simulink model "Speed_Controller_Test_gr3"  (Simulink 7.0)
settings: Solver=ode4  SolverMode=SingleTasking  StartTime=0.0  StopTime=252  FixedStep=0.01  RelTol=1e-3
InitFcn:
  | tempomat_para
StopFcn:
  | clear;
values from neighbouring files (symbols this model uses):
  A = 1.9    [tempomat_para.m]
  a_Fzg_max = 2    [tempomat_para.m]
  a_Fzg_min = -2    [tempomat_para.m]
  cw = 0.32    [tempomat_para.m]
  gang = [1 2 3 4]    [tempomat_para.m]
  gang_vec = [1 2 3 4]    [tempomat_para.m]
  i_anteil = 5    [tempomat_para.m]
  i_d = 3.42    [tempomat_para.m]
  i_g = [3.91 2.17 1.37 1.00]    [tempomat_para.m]
  lambda_gang = [1.3 1.25  1.17  1.05]    [tempomat_para.m]
  m_Fzg = 1400    [tempomat_para.m]
  M_mot_max = [130 149 163 170 168 166 162 158 150 139 123 80]    [tempomat_para.m]
  M_mot_min = [0 -40]    [tempomat_para.m]
  n_mot0 = 1000    [tempomat_para.m]
  n_mot_max = 1000:500:6500    [tempomat_para.m]
  n_mot_min = [1000 6500]    [tempomat_para.m]
  p_anteil = 100    [tempomat_para.m]
  r_dyn = 0.28    [tempomat_para.m]
  rho = 1.202    [tempomat_para.m]
  t_sch = 0.2    [tempomat_para.m]
  TI = [block '/TI']    [PSTI_callback.m]
  v_Fzg_ms0 = 0    [tempomat_para.m]
undefined symbols (not defined in the file or in its folder): Drossel_mat, getdatatypespecs
libraries: simulink x284, fzgbib x6
(part 15 of 19)

== system Speed_Controller_Test_gr3/Test Specification/R1 Speed Control step response/Maximum overshoot < 5 &  Steady state error < 5/Step response characteristics/Step response characteristics extraction/Extract steady state error ==
  Step response : Inport  OutDataType=sfix(16)  OutScaling=2^0
  Set point : Inport  Port=2  OutDataType=sfix(16)  OutScaling=2^0
  Subtract : Sum  Inputs=+-  OutDataType=sfix(16)  OutScaling=2^-10
  Weighted Moving Average : S-Function  FunctionName=sfix_fir  Parameters=(getdatatypespecs(OutDataType,OutScaling,DblOver,0)),[DoSatur RndMeth-1],DblOver,dolog,mgainval,(getdatatypespecs(GainDataType,GainScaling,DblOver,RadixGroup)),samptime,vinit,OutputDataTypeScalingMode,GainDataTypeScalingMode  mask(Weighted Moving Average){mgainval=0.01*ones(1,100), vinit=0.0, samptime=-1, GainDataTypeScalingMode=Inherit via internal rule, GainDataType=sfix( 16 ), MatRadixGroup=Best Precision: Matrix-wise, GainScaling=2^-10, OutputDataTypeScalingMode=Inherit via internal rule, OutDataType=sfix(16), OutScaling=2^-10, LockScale=off, RndMeth=Floor, DoSatur=off}
      mask prompts: mgainval "Weights:"; vinit "Initial condition:"; samptime "Sample time:"; GainDataTypeScalingMode "Gain data type and scaling:"; GainDataType "Parameter data type:     ex. sfix(16),  uint(8), float('single')"; MatRadixGroup "Parameter scaling mode:"; GainScaling "Parameter scaling:    Slope    ex.  2^-9"; OutputDataTypeScalingMode "Output data type and scaling:"; OutDataType "Output data type:     ex.  sfix(16),  uint(8),  float('single')"; OutScaling "Output scaling:    Slope or [Slope Bias]    ex.  2^-9"; LockScale "Lock output scaling so autoscaling tool can't change it"; RndMeth "Round toward:"; DoSatur "Saturate to max or min when overflows occur"
      mask help: Output the weighted moving average of the input.
      mask init:
      | DblOver = 0;
      | dolog = 0;
      | 
      | if MatRadixGroup == 5
      |     RadixGroup = 1; % BEST_PREC_MAT
      | elseif MatRadixGroup == 4
      |     RadixGroup = 2; % BEST_PREC_COL
      | elseif MatRadixGroup == 3
      |     RadixGroup = 3; % BEST_PREC_ROW
      | elseif MatRadixGroup == 2
      |     RadixGroup = 4; % BEST_PREC_ELE
      | else
      |     RadixGroup = 0; % BEST_PREC_OFF
      | end
      mask StyleString: edit,edit,edit,popup(Specify via dialog|Inherit via internal rule),edit,popup(Use Specified Scaling|Best Precision: Element-wise|Best Precision: Row-wise|Best Precision: Column-wise|Best Precision: Matrix-wise),edit,popup(Specify via dialog|Inherit via internal rule|Inherit via back propagation),edit,edit,checkbox,popup(Zero|Nearest|Ceiling|Floor),checkbox
      mask CallbackString: |||fixptdialog(gcbh)|fixptdialog(gcbh)|fixptdialog(gcbh)||fixptdialog(gcbh)|fixptdialog(gcbh)||||
      mask TabNameString: Main,Main,Main,Parameter data types,Parameter data types,Parameter data types,Parameter data types,Signal data types,Signal data types,Signal data types,Signal data types,Signal data types,Signal data types
      mask Display:
      | fprintf(fixpt_fir_mask_data(mgainval,'dispstr'))
      | plot(fixpt_fir_mask_data(mgainval,1),fixpt_fir_mask_data(mgainval,0))
  ss error : Outport  OutDataType=sfix(16)  OutScaling=2^0
  wires:
  Step response/1 -> Subtract/1
  Set point/1 -> Subtract/2
  Subtract/1 -> Weighted Moving Average/1
  Weighted Moving Average/1 -> ss error/1

== system Speed_Controller_Test_gr3/Test Specification/R1 Speed Control step response/Maximum overshoot < 5 &  Steady state error < 5/Step response characteristics/Step response characteristics extraction/Step time ==
  Clock : Inport  OutDataType=sfix(16)  OutScaling=2^0
  Trigger : TriggerPort
  Time : Outport  OutDataType=sfix(16)  OutScaling=2^0
  wires:
  Clock/1 -> Time/1

== system Speed_Controller_Test_gr3/Test Specification/R1 Speed Control step response/Maximum overshoot < 5 &  Steady state error < 5/Step response characteristics/Step response reset/Active if signals constant for some specified time ==
  Signal1 : Inport  OutDataType=sfix(16)  OutScaling=2^0
  Signal 2 : Inport  Port=2  OutDataType=sfix(16)  OutScaling=2^0
  Logical Operator1 : Logic  AllPortsSameDT=off  OutDataTypeMode=boolean
  Min Time : Constant  Value=10  OutDataType=sfix(16)  OutScaling=2^0
  MinMax : MinMax  Inputs=2  OutDataType=sfix(16)  OutScaling=2^0
  Relational Operator2 : RelationalOperator  Operator=<=  LogicOutDataTypeMode=boolean
  Switch : Switch  Criteria=u2 ~= 0
  Time since signal constant : Subsystem  TreatAsAtomicUnit=on  mask(Feature extraction block){RT=0.0001}
      mask prompts: RT "Relative tolerance in %"
      mask help: Detect if the signal value is constant (using the last two signal values) allowing for a user-defined relative deviation
      mask CallbackString:
      | if or( (str2double(get_param(gcb,'RT')) < 0), (str2double(get_param(gcb,'RT')) > 100))
      |     error(['Relative tolerance value (' get_param(gcb,'RT') ') out of range. Please give a value between 0 and 100.']);
      | else
      |     set_param([gcb '/Detect constant/Relative tolerance/Relative Tolerance'],'Value',get_param(gcb,'RT'));
      |     set_param([gcb '/Detect constant'],'RT',get_param(gcb,'RT'));
      | end
  Time since signal constant1 : Subsystem  TreatAsAtomicUnit=on  mask(Feature extraction block){RT=0.0001}
      mask prompts: RT "Relative tolerance in %"
      mask help: Detect if the signal value is constant (using the last two signal values) allowing for a user-defined relative deviation
      mask CallbackString:
      | if or( (str2double(get_param(gcb,'RT')) < 0), (str2double(get_param(gcb,'RT')) > 100))
      |     error(['Relative tolerance value (' get_param(gcb,'RT') ') out of range. Please give a value between 0 and 100.']);
      | else
      |     set_param([gcb '/Detect constant/Relative tolerance/Relative Tolerance'],'Value',get_param(gcb,'RT'));
      |     set_param([gcb '/Detect constant'],'RT',get_param(gcb,'RT'));
      | end
  Zero : Constant  Value=0  OutDataType=sfix(16)  OutScaling=2^0
  Constant signals : Outport  OutDataType=sfix(16)  OutScaling=2^0
  wires:
  Signal1/1 -> Time since signal constant/1(Signal)
  Signal 2/1 -> Time since signal constant1/1(Signal)
  Relational Operator2/1 -> Constant signals/1
  Min Time/1 -> Relational Operator2/1
  Switch/1 -> Relational Operator2/2
  Time since signal constant1/2(Feature) -> MinMax/2
  Time since signal constant/2(Feature) -> MinMax/1
  Time since signal constant/1(Trigger) -> Logical Operator1/1
  Time since signal constant1/1(Trigger) -> Logical Operator1/2
  MinMax/1 -> Switch/1
  Logical Operator1/1 -> Switch/2
  Zero/1 -> Switch/3

== system Speed_Controller_Test_gr3/Test Specification/R1 Speed Control step response/Maximum overshoot < 5 &  Steady state error < 5/Step response characteristics/Step response reset/Step detection ==
  Signal : Inport  OutDataType=sfix(16)  OutScaling=2^0
  Abs : Abs
  Add : Sum  Inputs=+-  OutDataType=sfix(16)  OutScaling=2^-10
  Clock : Clock
      settings: Decimation=10
  Memory : Memory
  Min step size : Constant  Value=10  OutDataType=sfix(16)  OutScaling=2^0
  Relational Operator : RelationalOperator  LogicOutDataTypeMode=boolean
  Switch : Switch  Criteria=u2 > Threshold
  Step : Outport  OutDataType=sfix(16)  OutScaling=2^0
  wires:
  Add/1 -> Abs/1
  Relational Operator/1 -> Step/1
  Min step size/1 -> Relational Operator/2
  Abs/1 -> Relational Operator/1
  Signal/1 -> Memory/1, Switch/3, Add/1
  Clock/1 -> Switch/2
  Memory/1 -> Switch/1
  Switch/1 -> Add/2

== system Speed_Controller_Test_gr3/Test Specification/R1 Speed Control step response/Maximum overshoot < 5 &  Steady state error < 5/Step response characteristics/Step response trigger/Active if signals constant for some specified time ==
  Signal1 : Inport  OutDataType=sfix(16)  OutScaling=2^0
  Signal 2 : Inport  Port=2  OutDataType=sfix(16)  OutScaling=2^0
  Logical Operator1 : Logic  AllPortsSameDT=off  OutDataTypeMode=boolean
  Min Time : Constant  Value=10  OutDataType=sfix(16)  OutScaling=2^0
  MinMax : MinMax  Inputs=2  OutDataType=sfix(16)  OutScaling=2^0
  Relational Operator2 : RelationalOperator  Operator=<=  LogicOutDataTypeMode=boolean
  Switch : Switch  Criteria=u2 ~= 0
  Time since signal constant : Subsystem  TreatAsAtomicUnit=on  mask(Feature extraction block){RT=0.001}
      mask prompts: RT "Relative tolerance in %"
      mask help: Detect if the signal value is constant (using the last two signal values) allowing for a user-defined relative deviation
      mask CallbackString:
      | if or( (str2double(get_param(gcb,'RT')) < 0), (str2double(get_param(gcb,'RT')) > 100))
      |     error(['Relative tolerance value (' get_param(gcb,'RT') ') out of range. Please give a value between 0 and 100.']);
      | else
      |     set_param([gcb '/Detect constant/Relative tolerance/Relative Tolerance'],'Value',get_param(gcb,'RT'));
      |     set_param([gcb '/Detect constant'],'RT',get_param(gcb,'RT'));
      | end
  Time since signal constant1 : Subsystem  TreatAsAtomicUnit=on  mask(Feature extraction block){RT=0.001}
      mask prompts: RT "Relative tolerance in %"
      mask help: Detect if the signal value is constant (using the last two signal values) allowing for a user-defined relative deviation
      mask CallbackString:
      | if or( (str2double(get_param(gcb,'RT')) < 0), (str2double(get_param(gcb,'RT')) > 100))
      |     error(['Relative tolerance value (' get_param(gcb,'RT') ') out of range. Please give a value between 0 and 100.']);
      | else
      |     set_param([gcb '/Detect constant/Relative tolerance/Relative Tolerance'],'Value',get_param(gcb,'RT'));
      |     set_param([gcb '/Detect constant'],'RT',get_param(gcb,'RT'));
      | end
  Zero : Constant  Value=0  OutDataType=sfix(16)  OutScaling=2^0
  Constant signals : Outport  OutDataType=sfix(16)  OutScaling=2^0
  wires:
  Signal1/1 -> Time since signal constant/1(Signal)
  Signal 2/1 -> Time since signal constant1/1(Signal)
  Relational Operator2/1 -> Constant signals/1
  Min Time/1 -> Relational Operator2/1
  Switch/1 -> Relational Operator2/2
  Time since signal constant1/2(Feature) -> MinMax/2
  Time since signal constant/2(Feature) -> MinMax/1
  Time since signal constant/1(Trigger) -> Logical Operator1/1
  Time since signal constant1/1(Trigger) -> Logical Operator1/2
  MinMax/1 -> Switch/1
  Logical Operator1/1 -> Switch/2
  Zero/1 -> Switch/3

== system Speed_Controller_Test_gr3/Test Specification/R1 Speed Control step response/Maximum overshoot < 5 &  Steady state error < 5/Step response characteristics/Step response trigger/Compare To Constant ==
  u : Inport  OutDataType=sfix(16)  OutScaling=2^0
  Compare : RelationalOperator  Operator=<=  LogicOutDataTypeMode=Specify via dialog  ZeroCross=off  InputSameDT=on
  Constant : Constant  Value=const  OutDataType=sfix(16)  OutScaling=1
  y : Outport  OutDataType=sfix(16)  OutScaling=2^0
  wires:
  Compare/1 -> y/1
  Constant/1 -> Compare/2
  u/1 -> Compare/1

== system Speed_Controller_Test_gr3/Test Specification/R1 Speed Control step response/Maximum overshoot < 5 &  Steady state error < 5/Step response characteristics/Step response trigger/Detect increase ==
  Signal : Inport  OutDataType=sfix(16)  OutScaling=2^0
  Clock : Clock
      settings: Decimation=10
  Memory : Memory
  Relational Operator : RelationalOperator  Operator=>  LogicOutDataTypeMode=Specify via dialog
  Switch : Switch  Criteria=u2 > Threshold
  Increase : Outport  OutDataType=sfix(16)  OutScaling=2^0
  wires:
  Switch/1 -> Relational Operator/2
  Memory/1 -> Switch/1
  Clock/1 -> Switch/2
  Relational Operator/1 -> Increase/1
  Signal/1 -> Switch/3, Memory/1, Relational Operator/1

== system Speed_Controller_Test_gr3/Test Specification/R2 Speed Control velocity restoration time after simple  acceleration/deceleration/CC active + no target & Speed Control active & step of V_Des = |1|  with time periods >= 7s/PS/TI/Delays1 ==
  In1 : Inport  OutDataType=sfix(16)  OutScaling=2^0
  Delay : Constant  Value=0  OutDataType=sfix(16)  OutScaling=2^0
  Integer Delay : S-Function  FunctionName=sfix_udelay  Parameters=samptime,vinit,NumDelays,1,1,0  mask(Integer Delay){vinit=0.0, samptime=-1, NumDelays=15}
      mask prompts: vinit "Initial condition:"; samptime "Sample time:"; NumDelays "Number of delays:"
      mask help: Delay a signal N sample periods.
      mask init:
      | if isempty(NumDelays)
      |    NumDelays = 1;
      | end
      mask Display: fprintf(' %d\nZ   ',-1*(NumDelays))
  Switch : Switch  Criteria=u2 ~= 0
  Out1 : Outport  OutDataType=sfix(16)  OutScaling=2^0
  wires:
  Switch/1 -> Out1/1
  In1/1 -> Switch/3, Integer Delay/1
  Delay/1 -> Switch/2
  Integer Delay/1 -> Switch/1

== system Speed_Controller_Test_gr3/Test Specification/R2 Speed Control velocity restoration time after simple  acceleration/deceleration/CC active + no target & Speed Control active & step of V_Des = |1|  with time periods >= 7s/PS/TI/Delays2 ==
  In1 : Inport  OutDataType=sfix(16)  OutScaling=2^0
  Delay : Constant  Value=0  OutDataType=sfix(16)  OutScaling=2^0
  Integer Delay : S-Function  FunctionName=sfix_udelay  Parameters=samptime,vinit,NumDelays,1,1,0  mask(Integer Delay){vinit=0.0, samptime=-1, NumDelays=15}
      mask prompts: vinit "Initial condition:"; samptime "Sample time:"; NumDelays "Number of delays:"
      mask help: Delay a signal N sample periods.
      mask init:
      | if isempty(NumDelays)
      |    NumDelays = 1;
      | end
      mask Display: fprintf(' %d\nZ   ',-1*(NumDelays))
  Switch : Switch  Criteria=u2 ~= 0
  Out1 : Outport  OutDataType=sfix(16)  OutScaling=2^0
  wires:
  Switch/1 -> Out1/1
  In1/1 -> Switch/3, Integer Delay/1
  Delay/1 -> Switch/2
  Integer Delay/1 -> Switch/1

== system Speed_Controller_Test_gr3/Test Specification/R2 Speed Control velocity restoration time after simple  acceleration/deceleration/CC active + no target & Speed Control active & step of V_Des = |1|  with time periods >= 7s/PS/TI/Delays3 ==
  In1 : Inport  OutDataType=sfix(16)  OutScaling=2^0
  Delay : Constant  Value=0  OutDataType=sfix(16)  OutScaling=2^0
  Integer Delay : S-Function  FunctionName=sfix_udelay  Parameters=samptime,vinit,NumDelays,1,1,0  mask(Integer Delay){vinit=0.0, samptime=-1, NumDelays=15}
      mask prompts: vinit "Initial condition:"; samptime "Sample time:"; NumDelays "Number of delays:"
      mask help: Delay a signal N sample periods.
      mask init:
      | if isempty(NumDelays)
      |    NumDelays = 1;
      | end
      mask Display: fprintf(' %d\nZ   ',-1*(NumDelays))
  Switch : Switch  Criteria=u2 ~= 0
  Out1 : Outport  OutDataType=sfix(16)  OutScaling=2^0
  wires:
  Switch/1 -> Out1/1
  In1/1 -> Switch/3, Integer Delay/1
  Delay/1 -> Switch/2
  Integer Delay/1 -> Switch/1

== system Speed_Controller_Test_gr3/Test Specification/R2 Speed Control velocity restoration time after simple  acceleration/deceleration/CC active + no target & Speed Control active & step of V_Des = |1|  with time periods >= 7s/PS/TID/Hold ==
  " " : Inport  OutDataType=sfix(16)  OutScaling=2^0
  "    " : Inport  Port=2  OutDataType=sfix(16)  OutScaling=2^0
  Memory : Memory  Orientation=left
  Switch : Switch  Criteria=u2 ~= 0
  "  " : Outport  OutDataType=sfix(16)  OutScaling=2^0
  wires:
  Memory/1 -> Switch/3
  Switch/1 -> Memory/1, "  "/1
  "    "/1 -> Switch/1
  " "/1 -> Switch/2

== system Speed_Controller_Test_gr3/Test Specification/R2 Speed Control velocity restoration time after simple  acceleration/deceleration/CC active + no target & Speed Control active & step of V_Des = |1|  with time periods >= 7s/Step with step size=|1|  and time periods >= 6s detection/Step detection/Active if signals constant for some specified time ==
  Signal 2 : Inport  OutDataType=sfix(16)  OutScaling=2^0
  Min Time : Constant  Value=6  OutDataType=sfix(16)  OutScaling=2^0
  Relational Operator2 : RelationalOperator  Operator=<=  LogicOutDataTypeMode=boolean
  Switch : Switch  Criteria=u2 ~= 0
  Time since signal constant1 : Subsystem  TreatAsAtomicUnit=on  mask(Feature extraction block){RT=0.0001}
      mask prompts: RT "Relative tolerance in %"
      mask help: Detect if the signal value is constant (using the last two signal values) allowing for a user-defined relative deviation
      mask CallbackString:
      | if or( (str2double(get_param(gcb,'RT')) < 0), (str2double(get_param(gcb,'RT')) > 100))
      |     error(['Relative tolerance value (' get_param(gcb,'RT') ') out of range. Please give a value between 0 and 100.']);
      | else
      |     set_param([gcb '/Detect constant/Relative tolerance/Relative Tolerance'],'Value',get_param(gcb,'RT'));
      |     set_param([gcb '/Detect constant'],'RT',get_param(gcb,'RT'));
      | end
  Zero : Constant  Value=0  OutDataType=sfix(16)  OutScaling=2^0
  Constant signals : Outport  OutDataType=sfix(16)  OutScaling=2^0
  wires:
  Signal 2/1 -> Time since signal constant1/1(Signal)
  Relational Operator2/1 -> Constant signals/1
  Min Time/1 -> Relational Operator2/1
  Switch/1 -> Relational Operator2/2
  Time since signal constant1/2(Feature) -> Switch/1
  Time since signal constant1/1(Trigger) -> Switch/2
  Zero/1 -> Switch/3

== system Speed_Controller_Test_gr3/Test Specification/R2 Speed Control velocity restoration time after simple  acceleration/deceleration/CC active + no target & Speed Control active & step of V_Des = |1|  with time periods >= 7s/Step with step size=|1|  and time periods >= 6s detection/Step detection/Step detection ==
  Signal : Inport  OutDataType=sfix(16)  OutScaling=2^0
  Abs : Abs
  Add : Sum  Inputs=+-  OutDataType=sfix(16)  OutScaling=2^-10
  Clock : Clock
      settings: Decimation=10
  Memory : Memory
  Relational Operator : RelationalOperator  Operator===  LogicOutDataTypeMode=boolean
  Step size : Constant  OutDataType=sfix(16)  OutScaling=2^0
  Switch : Switch  Criteria=u2 > Threshold
  Step : Outport  OutDataType=sfix(16)  OutScaling=2^0
  wires:
  Add/1 -> Abs/1
  Step size/1 -> Relational Operator/2
  Abs/1 -> Relational Operator/1
  Signal/1 -> Memory/1, Switch/3, Add/1
  Clock/1 -> Switch/2
  Memory/1 -> Switch/1
  Switch/1 -> Add/2
  Relational Operator/1 -> Step/1

== system Speed_Controller_Test_gr3/Test Specification/R2 Speed Control velocity restoration time after simple  acceleration/deceleration/after (6 seconds)  |V_Des-V_Vhcl <= 1.4|/PAS1/Delay bus signals/AD delay ==
  In1 : Inport  OutDataType=sfix(16)  OutScaling=2^0
  Delay : Constant  Value=0  OutDataType=sfix(16)  OutScaling=2^0
  Integer Delay : S-Function  FunctionName=sfix_udelay  Parameters=samptime,vinit,NumDelays,1,1,0  mask(Integer Delay){vinit=0.0, samptime=-1, NumDelays=15}
      mask prompts: vinit "Initial condition:"; samptime "Sample time:"; NumDelays "Number of delays:"
      mask help: Delay a signal N sample periods.
      mask init:
      | if isempty(NumDelays)
      |    NumDelays = 1;
      | end
      mask Display: fprintf(' %d\nZ   ',-1*(NumDelays))
  Switch : Switch  Criteria=u2 ~= 0
  Out1 : Outport  OutDataType=sfix(16)  OutScaling=2^0
  wires:
  Switch/1 -> Out1/1
  In1/1 -> Switch/3, Integer Delay/1
  Delay/1 -> Switch/2
  Integer Delay/1 -> Switch/1

== system Speed_Controller_Test_gr3/Test Specification/R2 Speed Control velocity restoration time after simple  acceleration/deceleration/after (6 seconds)  |V_Des-V_Vhcl <= 1.4|/PAS1/Delay bus signals/ELL delay ==
  In1 : Inport  OutDataType=sfix(16)  OutScaling=2^0
  Delay : Constant  Value=0  OutDataType=sfix(16)  OutScaling=2^0
  Integer Delay : S-Function  FunctionName=sfix_udelay  Parameters=samptime,vinit,NumDelays,1,1,0  mask(Integer Delay){vinit=0.0, samptime=-1, NumDelays=15}
      mask prompts: vinit "Initial condition:"; samptime "Sample time:"; NumDelays "Number of delays:"
      mask help: Delay a signal N sample periods.
      mask init:
      | if isempty(NumDelays)
      |    NumDelays = 1;
      | end
      mask Display: fprintf(' %d\nZ   ',-1*(NumDelays))
  Switch : Switch  Criteria=u2 ~= 0
  Out1 : Outport  OutDataType=sfix(16)  OutScaling=2^0
  wires:
  Switch/1 -> Out1/1
  In1/1 -> Switch/3, Integer Delay/1
  Delay/1 -> Switch/2
  Integer Delay/1 -> Switch/1

== system Speed_Controller_Test_gr3/Test Specification/R2 Speed Control velocity restoration time after simple  acceleration/deceleration/after (6 seconds)  |V_Des-V_Vhcl <= 1.4|/PAS1/Delay bus signals/EUL delay ==
  In1 : Inport  OutDataType=sfix(16)  OutScaling=2^0
  Delay : Constant  Value=0  OutDataType=sfix(16)  OutScaling=2^0
  Integer Delay : S-Function  FunctionName=sfix_udelay  Parameters=samptime,vinit,NumDelays,1,1,0  mask(Integer Delay){vinit=0.0, samptime=-1, NumDelays=15}
      mask prompts: vinit "Initial condition:"; samptime "Sample time:"; NumDelays "Number of delays:"
      mask help: Delay a signal N sample periods.
      mask init:
      | if isempty(NumDelays)
      |    NumDelays = 1;
      | end
      mask Display: fprintf(' %d\nZ   ',-1*(NumDelays))
  Switch : Switch  Criteria=u2 ~= 0
  Out1 : Outport  OutDataType=sfix(16)  OutScaling=2^0
  wires:
  Integer Delay/1 -> Switch/1
  Delay/1 -> Switch/2
  In1/1 -> Integer Delay/1, Switch/3
  Switch/1 -> Out1/1

== system Speed_Controller_Test_gr3/Test Specification/R2 Speed Control velocity restoration time after simple  acceleration/deceleration/after (6 seconds)  |V_Des-V_Vhcl <= 1.4|/PAS1/none - pass - fail/Arbitration ==
  Pass : Inport  OutDataType=sfix(16)  OutScaling=2^0
  Fail1 : Inport  Port=2  OutDataType=sfix(16)  OutScaling=2^0
  Fail2 : Inport  Port=3  OutDataType=sfix(16)  OutScaling=2^0
  Fail3 : Inport  Port=4  OutDataType=sfix(16)  OutScaling=2^0
  Fail4 : Inport  Port=5  OutDataType=sfix(16)  OutScaling=2^0
  Delay P F1 F3 : Inport  Port=6  OutDataType=sfix(16)  OutScaling=2^0
  Delay F2 : Inport  Port=7  OutDataType=sfix(16)  OutScaling=2^0
  Delay F4 : Inport  Port=8  OutDataType=sfix(16)  OutScaling=2^0
  Max delay : Inport  Port=9  OutDataType=sfix(16)  OutScaling=2^0
  Verdict identification : Subsystem
  Verdict selection : Subsystem
  Verdict : Outport  OutDataType=sfix(16)  OutScaling=2^0
  Delay : Outport  Port=2  OutDataType=sfix(16)  OutScaling=2^0
  wires:
  Verdict selection/2(Delay) -> Delay/1
  Verdict selection/1(Verdict) -> Verdict/1
  Max delay/1 -> Verdict selection/6(Max delay)
  Verdict identification/2(V2) -> Verdict selection/2(V2)
  Verdict identification/1(V1) -> Verdict selection/1(V1)
  Delay F4/1 -> Verdict selection/5(Delay F4)
  Delay F2/1 -> Verdict selection/4(Delay F2)
  Delay P F1 F3/1 -> Verdict selection/3(Delay P F1 F3)
  Fail4/1 -> Verdict identification/5(Fail4)
  Fail3/1 -> Verdict identification/4(Fail3)
  Fail2/1 -> Verdict identification/3(Fail2)
  Fail1/1 -> Verdict identification/2(Fail1)
  Pass/1 -> Verdict identification/1(Pass)

== system Speed_Controller_Test_gr3/Test Specification/R2 Speed Control velocity restoration time after simple  acceleration/deceleration/after (6 seconds)  |V_Des-V_Vhcl <= 1.4|/PAS1/none - pass - fail/Compute delay ==
  Max Delay : Inport  OutDataType=sfix(16)  OutScaling=2^0
  R AND : Inport  Port=2  OutDataType=sfix(16)  OutScaling=2^0
  Clock : Clock
      settings: Decimation=10
  Clock1 : Clock
      settings: Decimation=10
  Divide : Product  Inputs=/*  OutDataType=sfix(16)  OutScaling=2^-10
  Hold1 : Subsystem  TreatAsAtomicUnit=on
      mask Display: patch(-0.31+[0.4 0.46 0.46 0.54 0.54 0.6 0.6 0.55 0.55 0.45 0.45 0.4],-0.19+[0.85 0.85 0.95 0.95 0.85 0.85 0.87 0.87 0.96 0.96 0.87 0.87],[0 0 0]);
  SimStepSize : Constant  Value=0.01  OutDataType=sfix(16)  OutScaling=2^0
  Subtract : Sum  Inputs=-+  OutDataType=sfix(16)  OutScaling=2^-10
  Subtract1 : Sum  Inputs=+-  OutDataType=sfix(16)  OutScaling=2^-10
  Delay : Outport  OutDataType=sfix(16)  OutScaling=2^0
  wires:
  Divide/1 -> Delay/1
  Max Delay/1 -> Subtract/1
  SimStepSize/1 -> Divide/1
  Clock/1 -> Hold1/2("    ")
  Subtract/1 -> Subtract1/2
  Subtract1/1 -> Divide/2
  Clock1/1 -> Subtract1/1
  Hold1/1("  ") -> Subtract/2
  R AND/1 -> Hold1/1(" ")

== system Speed_Controller_Test_gr3/Test Specification/R2 Speed Control velocity restoration time after simple  acceleration/deceleration/after (6 seconds)  |V_Des-V_Vhcl <= 1.4|/PAS1/none - pass - fail/Compute delay1 ==
  Max Delay : Inport  OutDataType=sfix(16)  OutScaling=2^0
  R AND/z : Inport  Port=2  OutDataType=sfix(16)  OutScaling=2^0
  Add : Sum  OutDataType=sfix(16)  OutScaling=2^-10
  Clock : Clock
      settings: Decimation=10
  Clock1 : Clock
      settings: Decimation=10
  Divide : Product  Inputs=/*  OutDataType=sfix(16)  OutScaling=2^-10
  Hold1 : Subsystem  TreatAsAtomicUnit=on
      mask Display: patch(-0.31+[0.4 0.46 0.46 0.54 0.54 0.6 0.6 0.55 0.55 0.45 0.45 0.4],-0.19+[0.85 0.85 0.95 0.95 0.85 0.85 0.87 0.87 0.96 0.96 0.87 0.87],[0 0 0]);
  SimStepSize : Constant  Value=0.01  OutDataType=sfix(16)  OutScaling=2^0
  Subtract : Sum  Inputs=-+  OutDataType=sfix(16)  OutScaling=2^-10
  Subtract1 : Sum  Inputs=+-  OutDataType=sfix(16)  OutScaling=2^-10
  Unit : Constant  OutDataType=sfix(16)  OutScaling=2^0
  Delay : Outport  OutDataType=sfix(16)  OutScaling=2^0
  wires:
  Divide/1 -> Add/2
  Unit/1 -> Add/1
  Max Delay/1 -> Subtract/1
  SimStepSize/1 -> Divide/1
  Clock/1 -> Hold1/2("    ")
  Subtract/1 -> Subtract1/2
  Subtract1/1 -> Divide/2
  Clock1/1 -> Subtract1/1
  Hold1/1("  ") -> Subtract/2
  R AND/z/1 -> Hold1/1(" ")
  Add/1 -> Delay/1

== system Speed_Controller_Test_gr3/Test Specification/R2 Speed Control velocity restoration time after simple  acceleration/deceleration/after (6 seconds)  |V_Des-V_Vhcl <= 1.4|/PAS1/none - pass - fail/Compute delay2 ==
  Max Delay : Inport  OutDataType=sfix(16)  OutScaling=2^0
  Rp & NOT(Ra) : Inport  Port=2  OutDataType=sfix(16)  OutScaling=2^0
  Clock : Clock
      settings: Decimation=10
  Clock1 : Clock
      settings: Decimation=10
  Divide : Product  Inputs=/*  OutDataType=sfix(16)  OutScaling=2^-10
  Hold1 : Subsystem  TreatAsAtomicUnit=on
      mask Display: patch(-0.31+[0.4 0.46 0.46 0.54 0.54 0.6 0.6 0.55 0.55 0.45 0.45 0.4],-0.19+[0.85 0.85 0.95 0.95 0.85 0.85 0.87 0.87 0.96 0.96 0.87 0.87],[0 0 0]);
  SimStepSize : Constant  Value=0.01  OutDataType=sfix(16)  OutScaling=2^0
  Subtract : Sum  Inputs=-+  OutDataType=sfix(16)  OutScaling=2^-10
  Subtract1 : Sum  Inputs=+-  OutDataType=sfix(16)  OutScaling=2^-10
  Delay : Outport  OutDataType=sfix(16)  OutScaling=2^0
  wires:
  Divide/1 -> Delay/1
  Rp & NOT(Ra)/1 -> Hold1/1(" ")
  Hold1/1("  ") -> Subtract/2
  Clock1/1 -> Subtract1/1
  Subtract1/1 -> Divide/2
  Subtract/1 -> Subtract1/2
  Clock/1 -> Hold1/2("    ")
  SimStepSize/1 -> Divide/1
  Max Delay/1 -> Subtract/1

== system Speed_Controller_Test_gr3/Test Specification/R2 Speed Control velocity restoration time after simple  acceleration/deceleration/after (6 seconds)  |V_Des-V_Vhcl <= 1.4|/PAS1/none - pass - fail/Hold R AND1 ==
  " " : Inport  OutDataType=sfix(16)  OutScaling=2^0
  "    " : Inport  Port=2  OutDataType=sfix(16)  OutScaling=2^0
  Memory : Memory  Orientation=left
  Switch : Switch  Criteria=u2 ~= 0
  "  " : Outport  OutDataType=sfix(16)  OutScaling=2^0
  wires:
  Memory/1 -> Switch/3
  Switch/1 -> Memory/1, "  "/1
  "    "/1 -> Switch/1
  " "/1 -> Switch/2

== system Speed_Controller_Test_gr3/Test Specification/R2 Speed Control velocity restoration time after simple  acceleration/deceleration/after (6 seconds)  |V_Des-V_Vhcl <= 1.4|/PAS1/none - pass - fail/Hold R AND2 ==
  " " : Inport  OutDataType=sfix(16)  OutScaling=2^0
  "    " : Inport  Port=2  OutDataType=sfix(16)  OutScaling=2^0
  Memory : Memory  Orientation=left
  Switch : Switch  Criteria=u2 ~= 0
  "  " : Outport  OutDataType=sfix(16)  OutScaling=2^0
  wires:
  Memory/1 -> Switch/3
  Switch/1 -> Memory/1, "  "/1
  "    "/1 -> Switch/1
  " "/1 -> Switch/2

== system Speed_Controller_Test_gr3/Test Specification/R2 Speed Control velocity restoration time after simple  acceleration/deceleration/after (6 seconds)  |V_Des-V_Vhcl <= 1.4|/PAS1/none - pass - fail/Hold R AND3 ==
  " " : Inport  OutDataType=sfix(16)  OutScaling=2^0
  "    " : Inport  Port=2  OutDataType=sfix(16)  OutScaling=2^0
  Memory : Memory  Orientation=left
  Switch : Switch  Criteria=u2 ~= 0
  "  " : Outport  OutDataType=sfix(16)  OutScaling=2^0
  wires:
  " "/1 -> Switch/2
  "    "/1 -> Switch/1
  Switch/1 -> "  "/1, Memory/1
  Memory/1 -> Switch/3

== system Speed_Controller_Test_gr3/Test Specification/R2 Speed Control velocity restoration time after simple  acceleration/deceleration/after (6 seconds)  |V_Des-V_Vhcl <= 1.4|/PAS1/none - pass - fail/Hold1 ==
  " " : Inport  OutDataType=sfix(16)  OutScaling=2^0
  "    " : Inport  Port=2  OutDataType=sfix(16)  OutScaling=2^0
  Memory : Memory  Orientation=left
  Switch : Switch  Criteria=u2 ~= 0
  "  " : Outport  OutDataType=sfix(16)  OutScaling=2^0
  wires:
  Memory/1 -> Switch/3
  Switch/1 -> Memory/1, "  "/1
  "    "/1 -> Switch/1
  " "/1 -> Switch/2

== system Speed_Controller_Test_gr3/Test Specification/R2 Speed Control velocity restoration time after simple  acceleration/deceleration/after (6 seconds)  |V_Des-V_Vhcl <= 1.4|/PAS1/none - pass - fail/Hold2 ==
  " " : Inport  OutDataType=sfix(16)  OutScaling=2^0
  "    " : Inport  Port=2  OutDataType=sfix(16)  OutScaling=2^0
  Memory : Memory  Orientation=left
  Switch : Switch  Criteria=u2 ~= 0
  "  " : Outport  OutDataType=sfix(16)  OutScaling=2^0
  wires:
  Memory/1 -> Switch/3
  Switch/1 -> Memory/1, "  "/1
  "    "/1 -> Switch/1
  " "/1 -> Switch/2

== system Speed_Controller_Test_gr3/Test Specification/R2 Speed Control velocity restoration time after simple  acceleration/deceleration/after (6 seconds)  |V_Des-V_Vhcl <= 1.4|/PAS1/none - pass - fail/Hold3 ==
  " " : Inport  OutDataType=sfix(16)  OutScaling=2^0
  "    " : Inport  Port=2  OutDataType=sfix(16)  OutScaling=2^0
  Memory : Memory  Orientation=left
  Switch : Switch  Criteria=u2 ~= 0
  "  " : Outport  OutDataType=sfix(16)  OutScaling=2^0
  wires:
  " "/1 -> Switch/2
  "    "/1 -> Switch/1
  Switch/1 -> "  "/1, Memory/1
  Memory/1 -> Switch/3

== system Speed_Controller_Test_gr3/Test Specification/R2 Speed Control velocity restoration time after simple  acceleration/deceleration/after (6 seconds)  |V_Des-V_Vhcl <= 1.4|/PAS1/none - pass - fail/Hold4 ==
  " " : Inport  OutDataType=sfix(16)  OutScaling=2^0
  "    " : Inport  Port=2  OutDataType=sfix(16)  OutScaling=2^0
  Memory : Memory  Orientation=left
  Switch : Switch  Criteria=u2 ~= 0
  "  " : Outport  OutDataType=sfix(16)  OutScaling=2^0
  wires:
  Memory/1 -> Switch/3
  Switch/1 -> Memory/1, "  "/1
  "    "/1 -> Switch/1
  " "/1 -> Switch/2

== system Speed_Controller_Test_gr3/Test Specification/R2 Speed Control velocity restoration time after simple  acceleration/deceleration/after (6 seconds)  |V_Des-V_Vhcl <= 1.4|/PAS1/none - pass - fail/Hold5 ==
  " " : Inport  OutDataType=sfix(16)  OutScaling=2^0
  "    " : Inport  Port=2  OutDataType=sfix(16)  OutScaling=2^0
  Memory : Memory  Orientation=left
  Switch : Switch  Criteria=u2 ~= 0
  "  " : Outport  OutDataType=sfix(16)  OutScaling=2^0
  wires:
  " "/1 -> Switch/2
  "    "/1 -> Switch/1
  Switch/1 -> "  "/1, Memory/1
  Memory/1 -> Switch/3

== system Speed_Controller_Test_gr3/Test Specification/R2 Speed Control velocity restoration time after simple  acceleration/deceleration/after (6 seconds)  |V_Des-V_Vhcl <= 1.4|/PAS2/Delay bus signals/AD delay ==
  In1 : Inport  OutDataType=sfix(16)  OutScaling=2^0
  Delay : Constant  Value=0  OutDataType=sfix(16)  OutScaling=2^0
  Integer Delay : S-Function  FunctionName=sfix_udelay  Parameters=samptime,vinit,NumDelays,1,1,0  mask(Integer Delay){vinit=0.0, samptime=-1, NumDelays=15}
      mask prompts: vinit "Initial condition:"; samptime "Sample time:"; NumDelays "Number of delays:"
      mask help: Delay a signal N sample periods.
      mask init:
      | if isempty(NumDelays)
      |    NumDelays = 1;
      | end
      mask Display: fprintf(' %d\nZ   ',-1*(NumDelays))
  Switch : Switch  Criteria=u2 ~= 0
  Out1 : Outport  OutDataType=sfix(16)  OutScaling=2^0
  wires:
  Switch/1 -> Out1/1
  In1/1 -> Switch/3, Integer Delay/1
  Delay/1 -> Switch/2
  Integer Delay/1 -> Switch/1

== system Speed_Controller_Test_gr3/Test Specification/R2 Speed Control velocity restoration time after simple  acceleration/deceleration/after (6 seconds)  |V_Des-V_Vhcl <= 1.4|/PAS2/Delay bus signals/ELL delay ==
  In1 : Inport  OutDataType=sfix(16)  OutScaling=2^0
  Delay : Constant  Value=0  OutDataType=sfix(16)  OutScaling=2^0
  Integer Delay : S-Function  FunctionName=sfix_udelay  Parameters=samptime,vinit,NumDelays,1,1,0  mask(Integer Delay){vinit=0.0, samptime=-1, NumDelays=15}
      mask prompts: vinit "Initial condition:"; samptime "Sample time:"; NumDelays "Number of delays:"
      mask help: Delay a signal N sample periods.
      mask init:
      | if isempty(NumDelays)
      |    NumDelays = 1;
      | end
      mask Display: fprintf(' %d\nZ   ',-1*(NumDelays))
  Switch : Switch  Criteria=u2 ~= 0
  Out1 : Outport  OutDataType=sfix(16)  OutScaling=2^0
  wires:
  Switch/1 -> Out1/1
  In1/1 -> Switch/3, Integer Delay/1
  Delay/1 -> Switch/2
  Integer Delay/1 -> Switch/1

== system Speed_Controller_Test_gr3/Test Specification/R2 Speed Control velocity restoration time after simple  acceleration/deceleration/after (6 seconds)  |V_Des-V_Vhcl <= 1.4|/PAS2/Delay bus signals/EUL delay ==
  In1 : Inport  OutDataType=sfix(16)  OutScaling=2^0
  Delay : Constant  Value=0  OutDataType=sfix(16)  OutScaling=2^0
  Integer Delay : S-Function  FunctionName=sfix_udelay  Parameters=samptime,vinit,NumDelays,1,1,0  mask(Integer Delay){vinit=0.0, samptime=-1, NumDelays=15}
      mask prompts: vinit "Initial condition:"; samptime "Sample time:"; NumDelays "Number of delays:"
      mask help: Delay a signal N sample periods.
      mask init:
      | if isempty(NumDelays)
      |    NumDelays = 1;
      | end
      mask Display: fprintf(' %d\nZ   ',-1*(NumDelays))
  Switch : Switch  Criteria=u2 ~= 0
  Out1 : Outport  OutDataType=sfix(16)  OutScaling=2^0
  wires:
  Integer Delay/1 -> Switch/1
  Delay/1 -> Switch/2
  In1/1 -> Integer Delay/1, Switch/3
  Switch/1 -> Out1/1

== system Speed_Controller_Test_gr3/Test Specification/R2 Speed Control velocity restoration time after simple  acceleration/deceleration/after (6 seconds)  |V_Des-V_Vhcl <= 1.4|/PAS2/none - pass - fail/Arbitration ==
  Pass : Inport  OutDataType=sfix(16)  OutScaling=2^0
  Fail1 : Inport  Port=2  OutDataType=sfix(16)  OutScaling=2^0
  Fail2 : Inport  Port=3  OutDataType=sfix(16)  OutScaling=2^0
  Fail3 : Inport  Port=4  OutDataType=sfix(16)  OutScaling=2^0
  Fail4 : Inport  Port=5  OutDataType=sfix(16)  OutScaling=2^0
  Delay P F1 F3 : Inport  Port=6  OutDataType=sfix(16)  OutScaling=2^0
  Delay F2 : Inport  Port=7  OutDataType=sfix(16)  OutScaling=2^0
  Delay F4 : Inport  Port=8  OutDataType=sfix(16)  OutScaling=2^0
  Max delay : Inport  Port=9  OutDataType=sfix(16)  OutScaling=2^0
  Verdict identification : Subsystem
  Verdict selection : Subsystem
  Verdict : Outport  OutDataType=sfix(16)  OutScaling=2^0
  Delay : Outport  Port=2  OutDataType=sfix(16)  OutScaling=2^0
  wires:
  Verdict selection/2(Delay) -> Delay/1
  Verdict selection/1(Verdict) -> Verdict/1
  Max delay/1 -> Verdict selection/6(Max delay)
  Verdict identification/2(V2) -> Verdict selection/2(V2)
  Verdict identification/1(V1) -> Verdict selection/1(V1)
  Delay F4/1 -> Verdict selection/5(Delay F4)
  Delay F2/1 -> Verdict selection/4(Delay F2)
  Delay P F1 F3/1 -> Verdict selection/3(Delay P F1 F3)
  Fail4/1 -> Verdict identification/5(Fail4)
  Fail3/1 -> Verdict identification/4(Fail3)
  Fail2/1 -> Verdict identification/3(Fail2)
  Fail1/1 -> Verdict identification/2(Fail1)
  Pass/1 -> Verdict identification/1(Pass)

== system Speed_Controller_Test_gr3/Test Specification/R2 Speed Control velocity restoration time after simple  acceleration/deceleration/after (6 seconds)  |V_Des-V_Vhcl <= 1.4|/PAS2/none - pass - fail/Compute delay ==
  Max Delay : Inport  OutDataType=sfix(16)  OutScaling=2^0
  R AND : Inport  Port=2  OutDataType=sfix(16)  OutScaling=2^0
  Clock : Clock
      settings: Decimation=10
  Clock1 : Clock
      settings: Decimation=10
  Divide : Product  Inputs=/*  OutDataType=sfix(16)  OutScaling=2^-10
  Hold1 : Subsystem  TreatAsAtomicUnit=on
      mask Display: patch(-0.31+[0.4 0.46 0.46 0.54 0.54 0.6 0.6 0.55 0.55 0.45 0.45 0.4],-0.19+[0.85 0.85 0.95 0.95 0.85 0.85 0.87 0.87 0.96 0.96 0.87 0.87],[0 0 0]);
  SimStepSize : Constant  Value=0.01  OutDataType=sfix(16)  OutScaling=2^0
  Subtract : Sum  Inputs=-+  OutDataType=sfix(16)  OutScaling=2^-10
  Subtract1 : Sum  Inputs=+-  OutDataType=sfix(16)  OutScaling=2^-10
  Delay : Outport  OutDataType=sfix(16)  OutScaling=2^0
  wires:
  Divide/1 -> Delay/1
  Max Delay/1 -> Subtract/1
  SimStepSize/1 -> Divide/1
  Clock/1 -> Hold1/2("    ")
  Subtract/1 -> Subtract1/2
  Subtract1/1 -> Divide/2
  Clock1/1 -> Subtract1/1
  Hold1/1("  ") -> Subtract/2
  R AND/1 -> Hold1/1(" ")

== system Speed_Controller_Test_gr3/Test Specification/R2 Speed Control velocity restoration time after simple  acceleration/deceleration/after (6 seconds)  |V_Des-V_Vhcl <= 1.4|/PAS2/none - pass - fail/Compute delay1 ==
  Max Delay : Inport  OutDataType=sfix(16)  OutScaling=2^0
  R AND/z : Inport  Port=2  OutDataType=sfix(16)  OutScaling=2^0
  Add : Sum  OutDataType=sfix(16)  OutScaling=2^-10
  Clock : Clock
      settings: Decimation=10
  Clock1 : Clock
      settings: Decimation=10
  Divide : Product  Inputs=/*  OutDataType=sfix(16)  OutScaling=2^-10
  Hold1 : Subsystem  TreatAsAtomicUnit=on
      mask Display: patch(-0.31+[0.4 0.46 0.46 0.54 0.54 0.6 0.6 0.55 0.55 0.45 0.45 0.4],-0.19+[0.85 0.85 0.95 0.95 0.85 0.85 0.87 0.87 0.96 0.96 0.87 0.87],[0 0 0]);
  SimStepSize : Constant  Value=0.01  OutDataType=sfix(16)  OutScaling=2^0
  Subtract : Sum  Inputs=-+  OutDataType=sfix(16)  OutScaling=2^-10
  Subtract1 : Sum  Inputs=+-  OutDataType=sfix(16)  OutScaling=2^-10
  Unit : Constant  OutDataType=sfix(16)  OutScaling=2^0
  Delay : Outport  OutDataType=sfix(16)  OutScaling=2^0
  wires:
  Divide/1 -> Add/2
  Unit/1 -> Add/1
  Max Delay/1 -> Subtract/1
  SimStepSize/1 -> Divide/1
  Clock/1 -> Hold1/2("    ")
  Subtract/1 -> Subtract1/2
  Subtract1/1 -> Divide/2
  Clock1/1 -> Subtract1/1
  Hold1/1("  ") -> Subtract/2
  R AND/z/1 -> Hold1/1(" ")
  Add/1 -> Delay/1

== system Speed_Controller_Test_gr3/Test Specification/R2 Speed Control velocity restoration time after simple  acceleration/deceleration/after (6 seconds)  |V_Des-V_Vhcl <= 1.4|/PAS2/none - pass - fail/Compute delay2 ==
  Max Delay : Inport  OutDataType=sfix(16)  OutScaling=2^0
  Rp & NOT(Ra) : Inport  Port=2  OutDataType=sfix(16)  OutScaling=2^0
  Clock : Clock
      settings: Decimation=10
  Clock1 : Clock
      settings: Decimation=10
  Divide : Product  Inputs=/*  OutDataType=sfix(16)  OutScaling=2^-10
  Hold1 : Subsystem  TreatAsAtomicUnit=on
      mask Display: patch(-0.31+[0.4 0.46 0.46 0.54 0.54 0.6 0.6 0.55 0.55 0.45 0.45 0.4],-0.19+[0.85 0.85 0.95 0.95 0.85 0.85 0.87 0.87 0.96 0.96 0.87 0.87],[0 0 0]);
  SimStepSize : Constant  Value=0.01  OutDataType=sfix(16)  OutScaling=2^0
  Subtract : Sum  Inputs=-+  OutDataType=sfix(16)  OutScaling=2^-10
  Subtract1 : Sum  Inputs=+-  OutDataType=sfix(16)  OutScaling=2^-10
  Delay : Outport  OutDataType=sfix(16)  OutScaling=2^0
  wires:
  Divide/1 -> Delay/1
  Rp & NOT(Ra)/1 -> Hold1/1(" ")
  Hold1/1("  ") -> Subtract/2
  Clock1/1 -> Subtract1/1
  Subtract1/1 -> Divide/2
  Subtract/1 -> Subtract1/2
  Clock/1 -> Hold1/2("    ")
  SimStepSize/1 -> Divide/1
  Max Delay/1 -> Subtract/1

== system Speed_Controller_Test_gr3/Test Specification/R2 Speed Control velocity restoration time after simple  acceleration/deceleration/after (6 seconds)  |V_Des-V_Vhcl <= 1.4|/PAS2/none - pass - fail/Hold R AND1 ==
  " " : Inport  OutDataType=sfix(16)  OutScaling=2^0
  "    " : Inport  Port=2  OutDataType=sfix(16)  OutScaling=2^0
  Memory : Memory  Orientation=left
  Switch : Switch  Criteria=u2 ~= 0
  "  " : Outport  OutDataType=sfix(16)  OutScaling=2^0
  wires:
  Memory/1 -> Switch/3
  Switch/1 -> Memory/1, "  "/1
  "    "/1 -> Switch/1
  " "/1 -> Switch/2

== system Speed_Controller_Test_gr3/Test Specification/R2 Speed Control velocity restoration time after simple  acceleration/deceleration/after (6 seconds)  |V_Des-V_Vhcl <= 1.4|/PAS2/none - pass - fail/Hold R AND2 ==
  " " : Inport  OutDataType=sfix(16)  OutScaling=2^0
  "    " : Inport  Port=2  OutDataType=sfix(16)  OutScaling=2^0
  Memory : Memory  Orientation=left
  Switch : Switch  Criteria=u2 ~= 0
  "  " : Outport  OutDataType=sfix(16)  OutScaling=2^0
  wires:
  Memory/1 -> Switch/3
  Switch/1 -> Memory/1, "  "/1
  "    "/1 -> Switch/1
  " "/1 -> Switch/2

== system Speed_Controller_Test_gr3/Test Specification/R2 Speed Control velocity restoration time after simple  acceleration/deceleration/after (6 seconds)  |V_Des-V_Vhcl <= 1.4|/PAS2/none - pass - fail/Hold R AND3 ==
  " " : Inport  OutDataType=sfix(16)  OutScaling=2^0
  "    " : Inport  Port=2  OutDataType=sfix(16)  OutScaling=2^0
  Memory : Memory  Orientation=left
  Switch : Switch  Criteria=u2 ~= 0
  "  " : Outport  OutDataType=sfix(16)  OutScaling=2^0
  wires:
  " "/1 -> Switch/2
  "    "/1 -> Switch/1
  Switch/1 -> "  "/1, Memory/1
  Memory/1 -> Switch/3

== system Speed_Controller_Test_gr3/Test Specification/R2 Speed Control velocity restoration time after simple  acceleration/deceleration/after (6 seconds)  |V_Des-V_Vhcl <= 1.4|/PAS2/none - pass - fail/Hold1 ==
  " " : Inport  OutDataType=sfix(16)  OutScaling=2^0
  "    " : Inport  Port=2  OutDataType=sfix(16)  OutScaling=2^0
  Memory : Memory  Orientation=left
  Switch : Switch  Criteria=u2 ~= 0
  "  " : Outport  OutDataType=sfix(16)  OutScaling=2^0
  wires:
  Memory/1 -> Switch/3
  Switch/1 -> Memory/1, "  "/1
  "    "/1 -> Switch/1
  " "/1 -> Switch/2

== system Speed_Controller_Test_gr3/Test Specification/R2 Speed Control velocity restoration time after simple  acceleration/deceleration/after (6 seconds)  |V_Des-V_Vhcl <= 1.4|/PAS2/none - pass - fail/Hold2 ==
  " " : Inport  OutDataType=sfix(16)  OutScaling=2^0
  "    " : Inport  Port=2  OutDataType=sfix(16)  OutScaling=2^0
  Memory : Memory  Orientation=left
  Switch : Switch  Criteria=u2 ~= 0
  "  " : Outport  OutDataType=sfix(16)  OutScaling=2^0
  wires:
  Memory/1 -> Switch/3
  Switch/1 -> Memory/1, "  "/1
  "    "/1 -> Switch/1
  " "/1 -> Switch/2

== system Speed_Controller_Test_gr3/Test Specification/R2 Speed Control velocity restoration time after simple  acceleration/deceleration/after (6 seconds)  |V_Des-V_Vhcl <= 1.4|/PAS2/none - pass - fail/Hold3 ==
  " " : Inport  OutDataType=sfix(16)  OutScaling=2^0
  "    " : Inport  Port=2  OutDataType=sfix(16)  OutScaling=2^0
  Memory : Memory  Orientation=left
  Switch : Switch  Criteria=u2 ~= 0
  "  " : Outport  OutDataType=sfix(16)  OutScaling=2^0
  wires:
  " "/1 -> Switch/2
  "    "/1 -> Switch/1
  Switch/1 -> "  "/1, Memory/1
  Memory/1 -> Switch/3

== system Speed_Controller_Test_gr3/Test Specification/R2 Speed Control velocity restoration time after simple  acceleration/deceleration/after (6 seconds)  |V_Des-V_Vhcl <= 1.4|/PAS2/none - pass - fail/Hold4 ==
  " " : Inport  OutDataType=sfix(16)  OutScaling=2^0
  "    " : Inport  Port=2  OutDataType=sfix(16)  OutScaling=2^0
  Memory : Memory  Orientation=left
  Switch : Switch  Criteria=u2 ~= 0
  "  " : Outport  OutDataType=sfix(16)  OutScaling=2^0
  wires:
  Memory/1 -> Switch/3
  Switch/1 -> Memory/1, "  "/1
  "    "/1 -> Switch/1
  " "/1 -> Switch/2

== system Speed_Controller_Test_gr3/Test Specification/R2 Speed Control velocity restoration time after simple  acceleration/deceleration/after (6 seconds)  |V_Des-V_Vhcl <= 1.4|/PAS2/none - pass - fail/Hold5 ==
  " " : Inport  OutDataType=sfix(16)  OutScaling=2^0
  "    " : Inport  Port=2  OutDataType=sfix(16)  OutScaling=2^0
  Memory : Memory  Orientation=left
  Switch : Switch  Criteria=u2 ~= 0
  "  " : Outport  OutDataType=sfix(16)  OutScaling=2^0
  wires:
  " "/1 -> Switch/2
  "    "/1 -> Switch/1
  Switch/1 -> "  "/1, Memory/1
  Memory/1 -> Switch/3

== system Speed_Controller_Test_gr3/Test Specification/R2 Speed Control velocity restoration time after simple  acceleration/deceleration/after (6 seconds)  |V_Des-V_Vhcl <= 1.4|/R = 2/Active for  6s after R=1 /Time since R = 1 ==
  Signal : Inport  OutDataType=sfix(16)  OutScaling=2^0
  Clock : Clock
      settings: Decimation=10
  Logical Operator : Logic  Operator=NAND  AllPortsSameDT=off  OutDataTypeMode=boolean
  Logical Operator1 : Logic  Operator=NOT  AllPortsSameDT=off  OutDataTypeMode=boolean
  Memory : Memory  Orientation=left
  Memory1 : Memory
  R = 1 : Subsystem
  Subtract : Sum  Inputs=-+  OutDataType=sfix(16)  OutScaling=2^-10
  Switch : Switch  Criteria=u2 > Threshold
  Trigger : Outport  OutDataType=sfix(16)  OutScaling=2^0
  Feature : Outport  Port=2  OutDataType=sfix(16)  OutScaling=2^0
  wires:
  Logical Operator/1 -> Switch/2
  Logical Operator1/1 -> Logical Operator/2
  Memory1/1 -> Logical Operator1/1
  Memory/1 -> Switch/1
  Switch/1 -> Memory/1, Subtract/1
  Clock/1 -> Switch/3, Subtract/2
  Subtract/1 -> Feature/1
  R = 1/1(Out1) -> Memory1/1, Logical Operator/1, Trigger/1
  Signal/1 -> R = 1/1(In1)
